simulink model "ballAndPlate"  (R2018a)
settings: Solver=VariableStepAuto  StartTime=0.0  StopTime=25  RelTol=1e-3
libraries: simulink x1
settings Model: Creator=alexanderhiller  LastModifiedBy=alexanderhiller

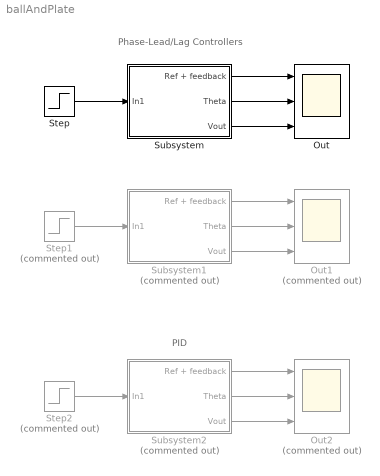
== system ballAndPlate ==
  note: Phase-Lead/Lag Controllers
  note: PID
  Out : Scope  NumInputPorts=3
  Out1 : Scope  Commented=on  NumInputPorts=3
  Out2 : Scope  Commented=on  NumInputPorts=3
  Step : Step  SampleTime=0
  Step1 : Step  Commented=on  SampleTime=0
  Step2 : Step  Commented=on  SampleTime=0
  Subsystem : Subsystem  mask{z_gc1=-14.7059, p_gc1=0, K_gc1=0.5, z_gc2=0, p_gc2=-1, K_gc2=0.5}
      mask prompts: z_gc1 "Zero of Gc1"; p_gc1 "Pole of Gc1"; K_gc1 "Gain of Gc1"; z_gc2 "Zero of Gc2"; p_gc2 "Pole of Gc2"; K_gc2 "Gain of Gc2"
  Subsystem1 : Subsystem  Commented=on  mask{z_gc1=-0.068, p_gc1=inf, K_gc1=1, z_gc2=0, p_gc2=0, K_gc2=0}
      mask prompts: z_gc1 "Zero of Gc1"; p_gc1 "Pole of Gc1"; K_gc1 "Gain of Gc1"; z_gc2 "Zero of Gc2"; p_gc2 "Pole of Gc2"; K_gc2 "Gain of Gc2"
  Subsystem2 : Subsystem  Commented=on  mask{z_gc1=-0.068, p_gc1=1, K_gc1=1}
      mask prompts: z_gc1 "Zero of Gc1"; p_gc1 "Pole of Gc1"; K_gc1 "Gain of Gc1"
  wires:
  Step/1 -> Subsystem/1(In1)
  Subsystem/1(Ref + feedback) -> Out/1
  Subsystem/2(Theta) -> Out/2
  Subsystem/3(Vout) -> Out/3
  Step1/1 -> Subsystem1/1(In1)
  Subsystem1/1(Ref + feedback) -> Out1/1
  Subsystem1/3(Vout) -> Out1/3
  Subsystem1/2(Theta) -> Out1/2
  Subsystem2/2(Theta) -> Out2/2
  Subsystem2/1(Ref + feedback) -> Out2/1
  Subsystem2/3(Vout) -> Out2/3
  Step2/1 -> Subsystem2/1(In1)

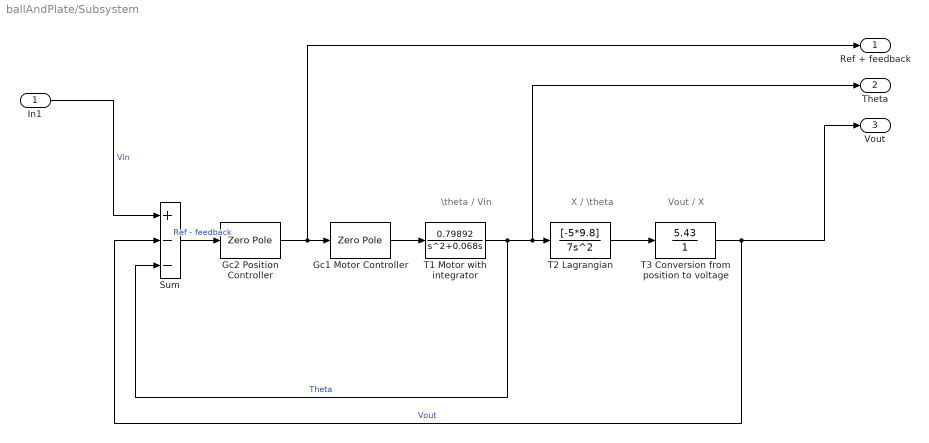
== system ballAndPlate/Subsystem ==
  note: \theta / Vin
  note: X / \theta
  note: Vout / X
  In1 : Inport
  Gc1 Motor Controller : ZeroPole  Zeros=[z_gc1]  Poles=[p_gc1]  Gain=[K_gc1]
  Gc2 Position Controller : ZeroPole  Zeros=[z_gc2]  Poles=[p_gc2]  Gain=[K_gc2]
  Sum : Sum  Inputs=+--
  "T1 Motor with integrator " : TransferFcn  Numerator=[0.79892]  Denominator=[1 0.068 0]
  "T2 Lagrangian " : TransferFcn  Numerator=[-5*9.8]  Denominator=[7 0 0]
  "T3 Conversion from position to voltage " : TransferFcn  Numerator=[5.43]  Denominator=[1]
  Ref + feedback : Outport
  Theta : Outport  Port=2
  Vout : Outport  Port=3
  wires:
  "T3 Conversion from position to voltage "/1 -> Vout/1, Sum/2  "Vout"
  In1/1 -> Sum/1  "Vin"
  Sum/1 -> Gc2 Position Controller/1  "Ref - feedback"
  "T2 Lagrangian "/1 -> "T3 Conversion from position to voltage "/1
  "T1 Motor with integrator "/1 -> Sum/3, Theta/1, "T2 Lagrangian "/1  "Theta"
  Gc2 Position Controller/1 -> Gc1 Motor Controller/1, Ref + feedback/1
  Gc1 Motor Controller/1 -> "T1 Motor with integrator "/1

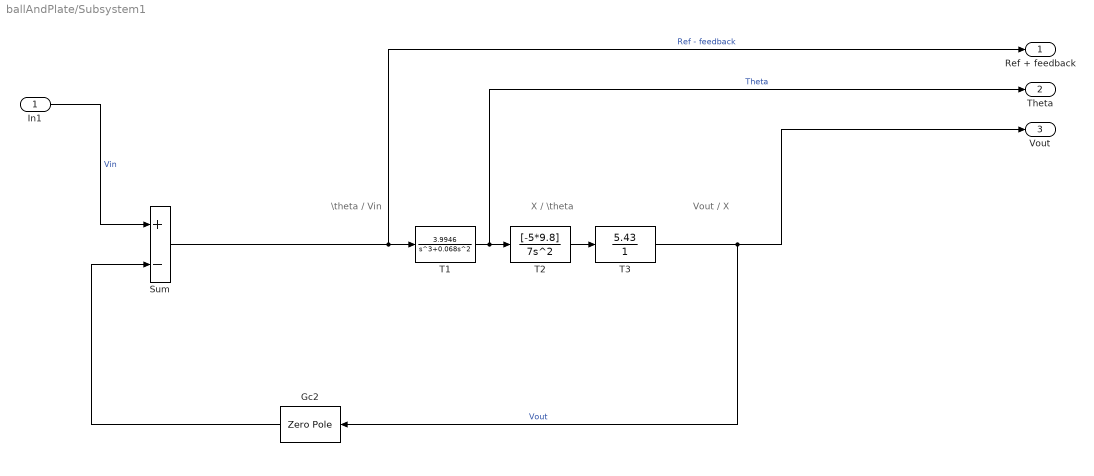
== system ballAndPlate/Subsystem1 ==
  note: \theta / Vin
  note: X / \theta
  note: Vout / X
  In1 : Inport
  Gc2 : ZeroPole  Zeros=[z_gc2]  Poles=[p_gc2]  Gain=[K_gc2]
  Sum : Sum  Inputs=+-
  "T1 " : TransferFcn  Numerator=[3.9946]  Denominator=[1 0.068 0 0]
  "T2 " : TransferFcn  Numerator=[-5*9.8]  Denominator=[7 0 0]
  "T3 " : TransferFcn  Numerator=[5.43]  Denominator=[1]
  Ref + feedback : Outport
  Theta : Outport  Port=2
  Vout : Outport  Port=3
  wires:
  "T3 "/1 -> Gc2/1, Vout/1  "Vout"
  In1/1 -> Sum/1  "Vin"
  Sum/1 -> Ref + feedback/1, "T1 "/1  "Ref - feedback"
  Gc2/1 -> Sum/2
  "T2 "/1 -> "T3 "/1
  "T1 "/1 -> Theta/1, "T2 "/1  "Theta"

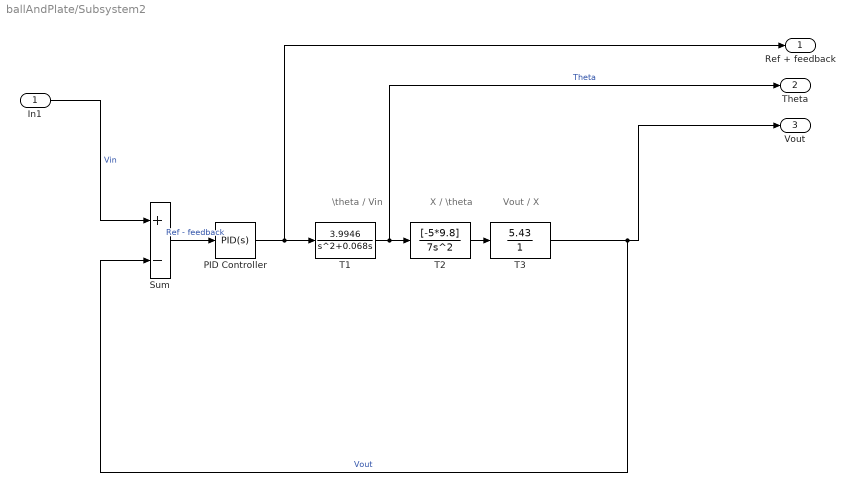
== system ballAndPlate/Subsystem2 ==
  note: \theta / Vin
  note: X / \theta
  note: Vout / X
  In1 : Inport
  PID Controller : simulink/Continuous/PID Controller  Controller=PID  TimeDomain=Continuous-time  SampleTime=-1  IntegratorMethod=Forward Euler  FilterMethod=Forward Euler  Form=Parallel  UseFilter=on  ControllerParametersSource=internal  P=1  I=1  D=0  N=100  InitialConditionSource=internal  InitialConditionForIntegrator=0  InitialConditionForFilter=0  ExternalReset=none  LimitOutput=off  UpperSaturationLimit=inf  LowerSaturationLimit=-inf  LinearizeAsGain=on  AntiWindupMode=none  Kb=1  TrackingMode=off  Kt=1  PParamMin=[]  PParamMax=[]  IParamMin=[]  IParamMax=[]  DParamMin=[]  DParamMax=[]  NParamMin=[]  NParamMax=[]  KbParamMin=[]  KbParamMax=[]  KtParamMin=[]  KtParamMax=[]  POutMin=[]  POutMax=[]  IOutMin=[]  IOutMax=[]  DOutMin=[]  DOutMax=[]  NOutMin=[]  NOutMax=[]  KbOutMin=[]  KbOutMax=[]  KtOutMin=[]  KtOutMax=[]  IntegratorOutMin=[]  IntegratorOutMax=[]  FilterOutMin=[]  FilterOutMax=[]  SumOutMin=[]  SumOutMax=[]  SumI1OutMin=[]  SumI1OutMax=[]  SumI2OutMin=[]  SumI2OutMax=[]  SumI3OutMin=[]  SumI3OutMax=[]  SumDOutMin=[]  SumDOutMax=[]  SaturationOutMin=[]  SaturationOutMax=[]  IntegratorContinuousStateAttributes=''  IntegratorStateMustResolveToSignalObject=off  IntegratorRTWStateStorageClass=Auto  FilterContinuousStateAttributes=''  FilterStateMustResolveToSignalObject=off  FilterRTWStateStorageClass=Auto  DifferentiatorICPrevScaledInput=0  DifferentiatorOutMin=[]  DifferentiatorOutMax=[]  FilterDiffOutCoefMin=[]  FilterDiffOutCoefMax=[]  SumDenOutMin=[]  SumDenOutMax=[]  SumNumOutMin=[]  SumNumOutMax=[]  ReciprocalOutMin=[]  ReciprocalOutMax=[]  DivideOutMin=[]  DivideOutMax=[]  TunerSelectOption=Transfer Function Based (PID Tuner App)
  Sum : Sum  Inputs=+-
  "T1 " : TransferFcn  Numerator=[3.9946]  Denominator=[1 0.068 0]
  "T2 " : TransferFcn  Numerator=[-5*9.8]  Denominator=[7 0 0]
  "T3 " : TransferFcn  Numerator=[5.43]  Denominator=[1]
  Ref + feedback : Outport
  Theta : Outport  Port=2
  Vout : Outport  Port=3
  wires:
  "T3 "/1 -> Sum/2, Vout/1  "Vout"
  In1/1 -> Sum/1  "Vin"
  Sum/1 -> PID Controller/1  "Ref - feedback"
  "T2 "/1 -> "T3 "/1
  "T1 "/1 -> Theta/1, "T2 "/1  "Theta"
  PID Controller/1 -> Ref + feedback/1, "T1 "/1
